simulink model "MySusp_FrcSystem_RTW"  (R2022a)
settings: Solver=ode1  StartTime=0.0  StopTime=inf  FixedStep=0.001  RelTol=1e-3
PreLoadFcn:
  | vehicle = 'Car'; if ~length(which('cmself')), cmenv; end
  | MySusp_FrcSystem_RTW_bus
  | MySusp_FrcSystem_RTW_params
InitFcn:
  | vehicle = 'Car'; if ~length(which('cmself')), cmenv; end
  | MySusp_FrcSystem_RTW_bus
undefined symbols (not defined in the file or in its folder): Damping_Pull_FL, Damping_Pull_FR, Damping_Pull_RL, Damping_Pull_RR, Damping_Push_FL, Damping_Push_FR, Damping_Push_RL, Damping_Push_RR, l0_Buffer_Pull_FL, l0_Buffer_Pull_FR, l0_Buffer_Pull_RL, l0_Buffer_Pull_RR, l0_Buffer_Push_FL, l0_Buffer_Push_FR, l0_Buffer_Push_RL, l0_Buffer_Push_RR, l0_Spring_FL, l0_Spring_FR, l0_Spring_RL, l0_Spring_RR, Stiffness_Buffer_Pull_FL, Stiffness_Buffer_Pull_FR, Stiffness_Buffer_Pull_RL, Stiffness_Buffer_Pull_RR, Stiffness_Buffer_Push_FL, Stiffness_Buffer_Push_FR, Stiffness_Buffer_Push_RL, Stiffness_Buffer_Push_RR, Stiffness_Spring_FL, Stiffness_Spring_FR, Stiffness_Spring_RL, Stiffness_Spring_RR, Stiffness_Stabi_F, Stiffness_Stabi_R
Description:
  | CarMaker Plug-in Model Target
settings Model: Creator=IPG  LastModifiedBy=IPG
settings SolverCC: AlgebraicLoopSolver=TrustRegion
settings DebuggingCC: UnconnectedInputMsg=warning  UnconnectedOutputMsg=warning  UnconnectedLineMsg=warning
settings RTWCC: Description=CarMaker Plug-in Model Target  SystemTargetFile=CarMaker.tlc  TemplateMakefile=CarMaker_unix-win64.tmf  DLArmComputeVersion=19.05
settings CodeAppCC: MaxIdLength=127
settings STFCustomTargetCC: TargetLangStandard=C99 (ISO)  CombineOutputUpdateFcns=on  CodeInterfacePackaging=Reusable function  GRTInterface=off  GenerateAllocFcn=on  SystemTargetFile=CarMaker.tlc
settings GRTTargetCC: ParMdlRefBuildCompliant=off  CompOptLevelCompliant=off  ConcurrentExecutionCompliant=off  MatFileLogging=off  CodeInterfacePackaging=Reusable function  CPPClassGenCompliant=off  GenerateAllocFcn=on  UseToolchainInfoCompliant=off

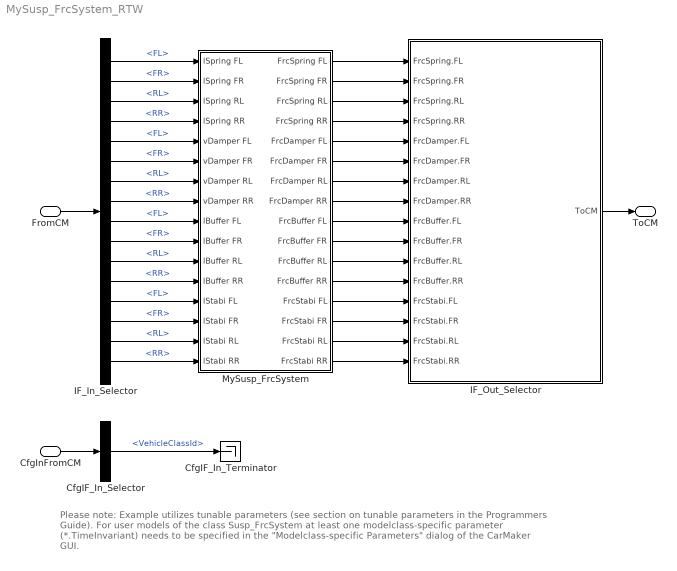
== system MySusp_FrcSystem_RTW ==
  note: Please note: Example utilizes tunable parameters (see section on tunable parameters in the Programmers Guide).
      |
      | For user models of the class Susp_FrcSystem at least one modelclass-specific parameter (*.TimeInvariant) needs to be
      | specified in the "Modelclass-specific Parameters" dialog of the CarMaker GUI.
  FromCM : Inport  OutDataTypeStr=Bus: cmSusp_FrcSystemIn
  CfgInFromCM : Inport  Port=2  OutDataTypeStr=Bus: cmSusp_FrcSystemCfgIn
  CfgIF_In_Selector : BusSelector  OutputSignals=VehicleClassId
  CfgIF_In_Terminator : Terminator
  IF_In_Selector : BusSelector  OutputSignals=lSpring.FL,lSpring.FR,lSpring.RL,lSpring.RR,vDamper.FL,vDamper.FR,vDamper.RL,vDamper.RR,lBuffer.FL,lBuffer.FR,lBuffer.RL,lBuffer.RR,lStabi.FL,lStabi.FR,lStabi.RL,lStabi.RR
  IF_Out_Selector : Subsystem  mask(Signal Selection){}
      mask help: Signal Selection Block
      settings: OpenFcn=cmSignalSelect('SignalSelection_CB',gcb)
  MySusp_FrcSystem : Subsystem
  ToCM : Outport  OutDataTypeStr=Bus: cmSusp_FrcSystemOut
  wires:
  FromCM/1 -> IF_In_Selector/1
  IF_Out_Selector/1(ToCM) -> ToCM/1
  CfgInFromCM/1 -> CfgIF_In_Selector/1
  CfgIF_In_Selector/1 -> CfgIF_In_Terminator/1  "<VehicleClassId>"
  MySusp_FrcSystem/1(FrcSpring FL) -> IF_Out_Selector/1(FrcSpring.FL)
  MySusp_FrcSystem/2(FrcSpring FR) -> IF_Out_Selector/2(FrcSpring.FR)
  MySusp_FrcSystem/3(FrcSpring RL) -> IF_Out_Selector/3(FrcSpring.RL)
  MySusp_FrcSystem/4(FrcSpring RR) -> IF_Out_Selector/4(FrcSpring.RR)
  MySusp_FrcSystem/5(FrcDamper FL) -> IF_Out_Selector/5(FrcDamper.FL)
  MySusp_FrcSystem/6(FrcDamper FR) -> IF_Out_Selector/6(FrcDamper.FR)
  MySusp_FrcSystem/7(FrcDamper RL) -> IF_Out_Selector/7(FrcDamper.RL)
  MySusp_FrcSystem/8(FrcDamper RR) -> IF_Out_Selector/8(FrcDamper.RR)
  MySusp_FrcSystem/9(FrcBuffer FL) -> IF_Out_Selector/9(FrcBuffer.FL)
  MySusp_FrcSystem/10(FrcBuffer FR) -> IF_Out_Selector/10(FrcBuffer.FR)
  MySusp_FrcSystem/11(FrcBuffer RL) -> IF_Out_Selector/11(FrcBuffer.RL)
  MySusp_FrcSystem/12(FrcBuffer RR) -> IF_Out_Selector/12(FrcBuffer.RR)
  MySusp_FrcSystem/13(FrcStabi FL) -> IF_Out_Selector/13(FrcStabi.FL)
  MySusp_FrcSystem/14(FrcStabi FR) -> IF_Out_Selector/14(FrcStabi.FR)
  MySusp_FrcSystem/15(FrcStabi RL) -> IF_Out_Selector/15(FrcStabi.RL)
  MySusp_FrcSystem/16(FrcStabi RR) -> IF_Out_Selector/16(FrcStabi.RR)
  IF_In_Selector/1 -> MySusp_FrcSystem/1(lSpring FL)  "<FL>"
  IF_In_Selector/2 -> MySusp_FrcSystem/2(lSpring FR)  "<FR>"
  IF_In_Selector/3 -> MySusp_FrcSystem/3(lSpring RL)  "<RL>"
  IF_In_Selector/4 -> MySusp_FrcSystem/4(lSpring RR)  "<RR>"
  IF_In_Selector/5 -> MySusp_FrcSystem/5(vDamper FL)  "<FL>"
  IF_In_Selector/6 -> MySusp_FrcSystem/6(vDamper FR)  "<FR>"
  IF_In_Selector/7 -> MySusp_FrcSystem/7(vDamper RL)  "<RL>"
  IF_In_Selector/8 -> MySusp_FrcSystem/8(vDamper RR)  "<RR>"
  IF_In_Selector/9 -> MySusp_FrcSystem/9(lBuffer FL)  "<FL>"
  IF_In_Selector/10 -> MySusp_FrcSystem/10(lBuffer FR)  "<FR>"
  IF_In_Selector/11 -> MySusp_FrcSystem/11(lBuffer RL)  "<RL>"
  IF_In_Selector/12 -> MySusp_FrcSystem/12(lBuffer RR)  "<RR>"
  IF_In_Selector/13 -> MySusp_FrcSystem/13(lStabi FL)  "<FL>"
  IF_In_Selector/14 -> MySusp_FrcSystem/14(lStabi FR)  "<FR>"
  IF_In_Selector/15 -> MySusp_FrcSystem/15(lStabi RL)  "<RL>"
  IF_In_Selector/16 -> MySusp_FrcSystem/16(lStabi RR)  "<RR>"

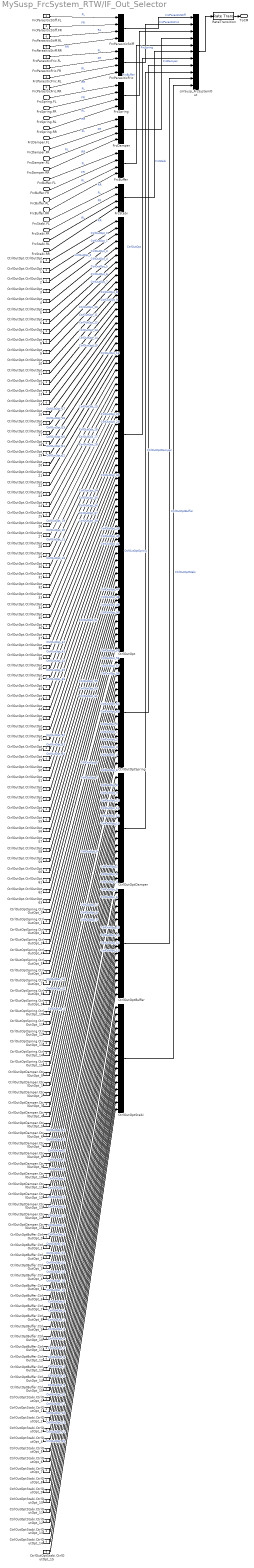
== system MySusp_FrcSystem_RTW/IF_Out_Selector ==
  FrcSpring.FL : Inport
  FrcSpring.FR : Inport  Port=2
  FrcSpring.RL : Inport  Port=3
  FrcSpring.RR : Inport  Port=4
  FrcDamper.FL : Inport  Port=5
  FrcDamper.FR : Inport  Port=6
  FrcDamper.RL : Inport  Port=7
  FrcDamper.RR : Inport  Port=8
  FrcBuffer.FL : Inport  Port=9
  FrcBuffer.FR : Inport  Port=10
  FrcBuffer.RL : Inport  Port=11
  FrcBuffer.RR : Inport  Port=12
  FrcStabi.FL : Inport  Port=13
  FrcStabi.FR : Inport  Port=14
  FrcStabi.RL : Inport  Port=15
  FrcStabi.RR : Inport  Port=16
  CtrlOutOpt : BusCreator  Inputs=64
  CtrlOutOpt.CtrlOutOpt_{0..63} (64 alike) : Constant  Value=0
  CtrlOutOptBuffer : BusCreator  Inputs=16
  CtrlOutOptBuffer.CtrlOutOpt_{0..15} (16 alike) : Constant  Value=0
  CtrlOutOptDamper : BusCreator  Inputs=16
  CtrlOutOptDamper.CtrlOutOpt_{0..15} (16 alike) : Constant  Value=0
  CtrlOutOptSpring : BusCreator  Inputs=16
  CtrlOutOptSpring.CtrlOutOpt_{0..15} (16 alike) : Constant  Value=0
  CtrlOutOptStabi : BusCreator  Inputs=16
  CtrlOutOptStabi.CtrlOutOpt_{0..15} (16 alike) : Constant  Value=0
  FrcBuffer : BusCreator  Inputs=4
  FrcDamper : BusCreator  Inputs=4
  FrcParasiticFric : BusCreator  Inputs=4
  FrcParasiticFric.FL : Constant  Value=0
  FrcParasiticFric.FR : Constant  Value=0
  FrcParasiticFric.RL : Constant  Value=0
  FrcParasiticFric.RR : Constant  Value=0
  FrcParasiticStiff : BusCreator  Inputs=4
  FrcParasiticStiff.FL : Constant  Value=0
  FrcParasiticStiff.FR : Constant  Value=0
  FrcParasiticStiff.RL : Constant  Value=0
  FrcParasiticStiff.RR : Constant  Value=0
  FrcSpring : BusCreator  Inputs=4
  FrcStabi : BusCreator  Inputs=4
  RateTransition : RateTransition  OutPortSampleTime=str2num(get_param(bdroot,'FixedStep'))
  cmSusp_FrcSystemOut : BusCreator  Inputs=11
  ToCM : Outport
  wires:
  RateTransition/1 -> ToCM/1
  cmSusp_FrcSystemOut/1 -> RateTransition/1
  FrcParasiticStiff/1 -> cmSusp_FrcSystemOut/1  "FrcParasiticStiff"
  FrcParasiticStiff.FL/1 -> FrcParasiticStiff/1  "FL"
  FrcParasiticStiff.FR/1 -> FrcParasiticStiff/2  "FR"
  FrcParasiticStiff.RL/1 -> FrcParasiticStiff/3  "RL"
  FrcParasiticStiff.RR/1 -> FrcParasiticStiff/4  "RR"
  FrcParasiticFric/1 -> cmSusp_FrcSystemOut/2  "FrcParasiticFric"
  FrcParasiticFric.FL/1 -> FrcParasiticFric/1  "FL"
  FrcParasiticFric.FR/1 -> FrcParasiticFric/2  "FR"
  FrcParasiticFric.RL/1 -> FrcParasiticFric/3  "RL"
  FrcParasiticFric.RR/1 -> FrcParasiticFric/4  "RR"
  FrcSpring/1 -> cmSusp_FrcSystemOut/3  "FrcSpring"
  FrcDamper/1 -> cmSusp_FrcSystemOut/4  "FrcDamper"
  FrcBuffer/1 -> cmSusp_FrcSystemOut/5  "FrcBuffer"
  FrcStabi/1 -> cmSusp_FrcSystemOut/6  "FrcStabi"
  CtrlOutOpt/1 -> cmSusp_FrcSystemOut/7  "CtrlOutOpt"
  CtrlOutOpt.CtrlOutOpt_0/1 -> CtrlOutOpt/1  "CtrlOutOpt_0"
  CtrlOutOpt.CtrlOutOpt_1/1 -> CtrlOutOpt/2  "CtrlOutOpt_1"
  CtrlOutOpt.CtrlOutOpt_2/1 -> CtrlOutOpt/3  "CtrlOutOpt_2"
  CtrlOutOpt.CtrlOutOpt_3/1 -> CtrlOutOpt/4  "CtrlOutOpt_3"
  CtrlOutOpt.CtrlOutOpt_4/1 -> CtrlOutOpt/5  "CtrlOutOpt_4"
  CtrlOutOpt.CtrlOutOpt_5/1 -> CtrlOutOpt/6  "CtrlOutOpt_5"
  CtrlOutOpt.CtrlOutOpt_6/1 -> CtrlOutOpt/7  "CtrlOutOpt_6"
  CtrlOutOpt.CtrlOutOpt_7/1 -> CtrlOutOpt/8  "CtrlOutOpt_7"
  CtrlOutOpt.CtrlOutOpt_8/1 -> CtrlOutOpt/9  "CtrlOutOpt_8"
  CtrlOutOpt.CtrlOutOpt_9/1 -> CtrlOutOpt/10  "CtrlOutOpt_9"
  CtrlOutOpt.CtrlOutOpt_10/1 -> CtrlOutOpt/11  "CtrlOutOpt_10"
  CtrlOutOpt.CtrlOutOpt_11/1 -> CtrlOutOpt/12  "CtrlOutOpt_11"
  CtrlOutOpt.CtrlOutOpt_12/1 -> CtrlOutOpt/13  "CtrlOutOpt_12"
  CtrlOutOpt.CtrlOutOpt_13/1 -> CtrlOutOpt/14  "CtrlOutOpt_13"
  CtrlOutOpt.CtrlOutOpt_14/1 -> CtrlOutOpt/15  "CtrlOutOpt_14"
  CtrlOutOpt.CtrlOutOpt_15/1 -> CtrlOutOpt/16  "CtrlOutOpt_15"
  CtrlOutOpt.CtrlOutOpt_16/1 -> CtrlOutOpt/17  "CtrlOutOpt_16"
  CtrlOutOpt.CtrlOutOpt_17/1 -> CtrlOutOpt/18  "CtrlOutOpt_17"
  CtrlOutOpt.CtrlOutOpt_18/1 -> CtrlOutOpt/19  "CtrlOutOpt_18"
  CtrlOutOpt.CtrlOutOpt_19/1 -> CtrlOutOpt/20  "CtrlOutOpt_19"
  CtrlOutOpt.CtrlOutOpt_20/1 -> CtrlOutOpt/21  "CtrlOutOpt_20"
  CtrlOutOpt.CtrlOutOpt_21/1 -> CtrlOutOpt/22  "CtrlOutOpt_21"
  CtrlOutOpt.CtrlOutOpt_22/1 -> CtrlOutOpt/23  "CtrlOutOpt_22"
  CtrlOutOpt.CtrlOutOpt_23/1 -> CtrlOutOpt/24  "CtrlOutOpt_23"
  CtrlOutOpt.CtrlOutOpt_24/1 -> CtrlOutOpt/25  "CtrlOutOpt_24"
  CtrlOutOpt.CtrlOutOpt_25/1 -> CtrlOutOpt/26  "CtrlOutOpt_25"
  CtrlOutOpt.CtrlOutOpt_26/1 -> CtrlOutOpt/27  "CtrlOutOpt_26"
  CtrlOutOpt.CtrlOutOpt_27/1 -> CtrlOutOpt/28  "CtrlOutOpt_27"
  CtrlOutOpt.CtrlOutOpt_28/1 -> CtrlOutOpt/29  "CtrlOutOpt_28"
  CtrlOutOpt.CtrlOutOpt_29/1 -> CtrlOutOpt/30  "CtrlOutOpt_29"
  CtrlOutOpt.CtrlOutOpt_30/1 -> CtrlOutOpt/31  "CtrlOutOpt_30"
  CtrlOutOpt.CtrlOutOpt_31/1 -> CtrlOutOpt/32  "CtrlOutOpt_31"
  CtrlOutOpt.CtrlOutOpt_32/1 -> CtrlOutOpt/33  "CtrlOutOpt_32"
  CtrlOutOpt.CtrlOutOpt_33/1 -> CtrlOutOpt/34  "CtrlOutOpt_33"
  CtrlOutOpt.CtrlOutOpt_34/1 -> CtrlOutOpt/35  "CtrlOutOpt_34"
  CtrlOutOpt.CtrlOutOpt_35/1 -> CtrlOutOpt/36  "CtrlOutOpt_35"
  CtrlOutOpt.CtrlOutOpt_36/1 -> CtrlOutOpt/37  "CtrlOutOpt_36"
  CtrlOutOpt.CtrlOutOpt_37/1 -> CtrlOutOpt/38  "CtrlOutOpt_37"
  CtrlOutOpt.CtrlOutOpt_38/1 -> CtrlOutOpt/39  "CtrlOutOpt_38"
  CtrlOutOpt.CtrlOutOpt_39/1 -> CtrlOutOpt/40  "CtrlOutOpt_39"
  CtrlOutOpt.CtrlOutOpt_40/1 -> CtrlOutOpt/41  "CtrlOutOpt_40"
  CtrlOutOpt.CtrlOutOpt_41/1 -> CtrlOutOpt/42  "CtrlOutOpt_41"
  CtrlOutOpt.CtrlOutOpt_42/1 -> CtrlOutOpt/43  "CtrlOutOpt_42"
  CtrlOutOpt.CtrlOutOpt_43/1 -> CtrlOutOpt/44  "CtrlOutOpt_43"
  CtrlOutOpt.CtrlOutOpt_44/1 -> CtrlOutOpt/45  "CtrlOutOpt_44"
  CtrlOutOpt.CtrlOutOpt_45/1 -> CtrlOutOpt/46  "CtrlOutOpt_45"
  CtrlOutOpt.CtrlOutOpt_46/1 -> CtrlOutOpt/47  "CtrlOutOpt_46"
  CtrlOutOpt.CtrlOutOpt_47/1 -> CtrlOutOpt/48  "CtrlOutOpt_47"
  CtrlOutOpt.CtrlOutOpt_48/1 -> CtrlOutOpt/49  "CtrlOutOpt_48"
  CtrlOutOpt.CtrlOutOpt_49/1 -> CtrlOutOpt/50  "CtrlOutOpt_49"
  CtrlOutOpt.CtrlOutOpt_50/1 -> CtrlOutOpt/51  "CtrlOutOpt_50"
  CtrlOutOpt.CtrlOutOpt_51/1 -> CtrlOutOpt/52  "CtrlOutOpt_51"
  CtrlOutOpt.CtrlOutOpt_52/1 -> CtrlOutOpt/53  "CtrlOutOpt_52"
  CtrlOutOpt.CtrlOutOpt_53/1 -> CtrlOutOpt/54  "CtrlOutOpt_53"
  CtrlOutOpt.CtrlOutOpt_54/1 -> CtrlOutOpt/55  "CtrlOutOpt_54"
  CtrlOutOpt.CtrlOutOpt_55/1 -> CtrlOutOpt/56  "CtrlOutOpt_55"
  CtrlOutOpt.CtrlOutOpt_56/1 -> CtrlOutOpt/57  "CtrlOutOpt_56"
  CtrlOutOpt.CtrlOutOpt_57/1 -> CtrlOutOpt/58  "CtrlOutOpt_57"
  CtrlOutOpt.CtrlOutOpt_58/1 -> CtrlOutOpt/59  "CtrlOutOpt_58"
  CtrlOutOpt.CtrlOutOpt_59/1 -> CtrlOutOpt/60  "CtrlOutOpt_59"
  CtrlOutOpt.CtrlOutOpt_60/1 -> CtrlOutOpt/61  "CtrlOutOpt_60"
  CtrlOutOpt.CtrlOutOpt_61/1 -> CtrlOutOpt/62  "CtrlOutOpt_61"
  CtrlOutOpt.CtrlOutOpt_62/1 -> CtrlOutOpt/63  "CtrlOutOpt_62"
  CtrlOutOpt.CtrlOutOpt_63/1 -> CtrlOutOpt/64  "CtrlOutOpt_63"
  CtrlOutOptSpring/1 -> cmSusp_FrcSystemOut/8  "CtrlOutOptSpring"
  CtrlOutOptSpring.CtrlOutOpt_0/1 -> CtrlOutOptSpring/1  "CtrlOutOpt_0"
  CtrlOutOptSpring.CtrlOutOpt_1/1 -> CtrlOutOptSpring/2  "CtrlOutOpt_1"
  CtrlOutOptSpring.CtrlOutOpt_2/1 -> CtrlOutOptSpring/3  "CtrlOutOpt_2"
  CtrlOutOptSpring.CtrlOutOpt_3/1 -> CtrlOutOptSpring/4  "CtrlOutOpt_3"
  CtrlOutOptSpring.CtrlOutOpt_4/1 -> CtrlOutOptSpring/5  "CtrlOutOpt_4"
  CtrlOutOptSpring.CtrlOutOpt_5/1 -> CtrlOutOptSpring/6  "CtrlOutOpt_5"
  CtrlOutOptSpring.CtrlOutOpt_6/1 -> CtrlOutOptSpring/7  "CtrlOutOpt_6"
  CtrlOutOptSpring.CtrlOutOpt_7/1 -> CtrlOutOptSpring/8  "CtrlOutOpt_7"
  CtrlOutOptSpring.CtrlOutOpt_8/1 -> CtrlOutOptSpring/9  "CtrlOutOpt_8"
  CtrlOutOptSpring.CtrlOutOpt_9/1 -> CtrlOutOptSpring/10  "CtrlOutOpt_9"
  CtrlOutOptSpring.CtrlOutOpt_10/1 -> CtrlOutOptSpring/11  "CtrlOutOpt_10"
  CtrlOutOptSpring.CtrlOutOpt_11/1 -> CtrlOutOptSpring/12  "CtrlOutOpt_11"
  CtrlOutOptSpring.CtrlOutOpt_12/1 -> CtrlOutOptSpring/13  "CtrlOutOpt_12"
  CtrlOutOptSpring.CtrlOutOpt_13/1 -> CtrlOutOptSpring/14  "CtrlOutOpt_13"
  CtrlOutOptSpring.CtrlOutOpt_14/1 -> CtrlOutOptSpring/15  "CtrlOutOpt_14"
  CtrlOutOptSpring.CtrlOutOpt_15/1 -> CtrlOutOptSpring/16  "CtrlOutOpt_15"
  CtrlOutOptDamper/1 -> cmSusp_FrcSystemOut/9  "CtrlOutOptDamper"
  CtrlOutOptDamper.CtrlOutOpt_0/1 -> CtrlOutOptDamper/1  "CtrlOutOpt_0"
  CtrlOutOptDamper.CtrlOutOpt_1/1 -> CtrlOutOptDamper/2  "CtrlOutOpt_1"
  CtrlOutOptDamper.CtrlOutOpt_2/1 -> CtrlOutOptDamper/3  "CtrlOutOpt_2"
  CtrlOutOptDamper.CtrlOutOpt_3/1 -> CtrlOutOptDamper/4  "CtrlOutOpt_3"
  CtrlOutOptDamper.CtrlOutOpt_4/1 -> CtrlOutOptDamper/5  "CtrlOutOpt_4"
  CtrlOutOptDamper.CtrlOutOpt_5/1 -> CtrlOutOptDamper/6  "CtrlOutOpt_5"
  CtrlOutOptDamper.CtrlOutOpt_6/1 -> CtrlOutOptDamper/7  "CtrlOutOpt_6"
  CtrlOutOptDamper.CtrlOutOpt_7/1 -> CtrlOutOptDamper/8  "CtrlOutOpt_7"
  CtrlOutOptDamper.CtrlOutOpt_8/1 -> CtrlOutOptDamper/9  "CtrlOutOpt_8"
  CtrlOutOptDamper.CtrlOutOpt_9/1 -> CtrlOutOptDamper/10  "CtrlOutOpt_9"
  CtrlOutOptDamper.CtrlOutOpt_10/1 -> CtrlOutOptDamper/11  "CtrlOutOpt_10"
  CtrlOutOptDamper.CtrlOutOpt_11/1 -> CtrlOutOptDamper/12  "CtrlOutOpt_11"
  CtrlOutOptDamper.CtrlOutOpt_12/1 -> CtrlOutOptDamper/13  "CtrlOutOpt_12"
  CtrlOutOptDamper.CtrlOutOpt_13/1 -> CtrlOutOptDamper/14  "CtrlOutOpt_13"
  CtrlOutOptDamper.CtrlOutOpt_14/1 -> CtrlOutOptDamper/15  "CtrlOutOpt_14"
  CtrlOutOptDamper.CtrlOutOpt_15/1 -> CtrlOutOptDamper/16  "CtrlOutOpt_15"
  CtrlOutOptBuffer/1 -> cmSusp_FrcSystemOut/10  "CtrlOutOptBuffer"
  CtrlOutOptBuffer.CtrlOutOpt_0/1 -> CtrlOutOptBuffer/1  "CtrlOutOpt_0"
  CtrlOutOptBuffer.CtrlOutOpt_1/1 -> CtrlOutOptBuffer/2  "CtrlOutOpt_1"
  CtrlOutOptBuffer.CtrlOutOpt_2/1 -> CtrlOutOptBuffer/3  "CtrlOutOpt_2"
  CtrlOutOptBuffer.CtrlOutOpt_3/1 -> CtrlOutOptBuffer/4  "CtrlOutOpt_3"
  CtrlOutOptBuffer.CtrlOutOpt_4/1 -> CtrlOutOptBuffer/5  "CtrlOutOpt_4"
  CtrlOutOptBuffer.CtrlOutOpt_5/1 -> CtrlOutOptBuffer/6  "CtrlOutOpt_5"
  CtrlOutOptBuffer.CtrlOutOpt_6/1 -> CtrlOutOptBuffer/7  "CtrlOutOpt_6"
  CtrlOutOptBuffer.CtrlOutOpt_7/1 -> CtrlOutOptBuffer/8  "CtrlOutOpt_7"
  CtrlOutOptBuffer.CtrlOutOpt_8/1 -> CtrlOutOptBuffer/9  "CtrlOutOpt_8"
  CtrlOutOptBuffer.CtrlOutOpt_9/1 -> CtrlOutOptBuffer/10  "CtrlOutOpt_9"
  CtrlOutOptBuffer.CtrlOutOpt_10/1 -> CtrlOutOptBuffer/11  "CtrlOutOpt_10"
  CtrlOutOptBuffer.CtrlOutOpt_11/1 -> CtrlOutOptBuffer/12  "CtrlOutOpt_11"
  CtrlOutOptBuffer.CtrlOutOpt_12/1 -> CtrlOutOptBuffer/13  "CtrlOutOpt_12"
  CtrlOutOptBuffer.CtrlOutOpt_13/1 -> CtrlOutOptBuffer/14  "CtrlOutOpt_13"
  CtrlOutOptBuffer.CtrlOutOpt_14/1 -> CtrlOutOptBuffer/15  "CtrlOutOpt_14"
  CtrlOutOptBuffer.CtrlOutOpt_15/1 -> CtrlOutOptBuffer/16  "CtrlOutOpt_15"
  CtrlOutOptStabi/1 -> cmSusp_FrcSystemOut/11  "CtrlOutOptStabi"
  CtrlOutOptStabi.CtrlOutOpt_0/1 -> CtrlOutOptStabi/1  "CtrlOutOpt_0"
  CtrlOutOptStabi.CtrlOutOpt_1/1 -> CtrlOutOptStabi/2  "CtrlOutOpt_1"
  CtrlOutOptStabi.CtrlOutOpt_2/1 -> CtrlOutOptStabi/3  "CtrlOutOpt_2"
  CtrlOutOptStabi.CtrlOutOpt_3/1 -> CtrlOutOptStabi/4  "CtrlOutOpt_3"
  CtrlOutOptStabi.CtrlOutOpt_4/1 -> CtrlOutOptStabi/5  "CtrlOutOpt_4"
  CtrlOutOptStabi.CtrlOutOpt_5/1 -> CtrlOutOptStabi/6  "CtrlOutOpt_5"
  CtrlOutOptStabi.CtrlOutOpt_6/1 -> CtrlOutOptStabi/7  "CtrlOutOpt_6"
  CtrlOutOptStabi.CtrlOutOpt_7/1 -> CtrlOutOptStabi/8  "CtrlOutOpt_7"
  CtrlOutOptStabi.CtrlOutOpt_8/1 -> CtrlOutOptStabi/9  "CtrlOutOpt_8"
  CtrlOutOptStabi.CtrlOutOpt_9/1 -> CtrlOutOptStabi/10  "CtrlOutOpt_9"
  CtrlOutOptStabi.CtrlOutOpt_10/1 -> CtrlOutOptStabi/11  "CtrlOutOpt_10"
  CtrlOutOptStabi.CtrlOutOpt_11/1 -> CtrlOutOptStabi/12  "CtrlOutOpt_11"
  CtrlOutOptStabi.CtrlOutOpt_12/1 -> CtrlOutOptStabi/13  "CtrlOutOpt_12"
  CtrlOutOptStabi.CtrlOutOpt_13/1 -> CtrlOutOptStabi/14  "CtrlOutOpt_13"
  CtrlOutOptStabi.CtrlOutOpt_14/1 -> CtrlOutOptStabi/15  "CtrlOutOpt_14"
  CtrlOutOptStabi.CtrlOutOpt_15/1 -> CtrlOutOptStabi/16  "CtrlOutOpt_15"
  FrcSpring.FL/1 -> FrcSpring/1  "FL"
  FrcSpring.FR/1 -> FrcSpring/2  "FR"
  FrcSpring.RL/1 -> FrcSpring/3  "RL"
  FrcSpring.RR/1 -> FrcSpring/4  "RR"
  FrcDamper.FL/1 -> FrcDamper/1  "FL"
  FrcDamper.FR/1 -> FrcDamper/2  "FR"
  FrcDamper.RL/1 -> FrcDamper/3  "RL"
  FrcDamper.RR/1 -> FrcDamper/4  "RR"
  FrcBuffer.FL/1 -> FrcBuffer/1  "FL"
  FrcBuffer.FR/1 -> FrcBuffer/2  "FR"
  FrcBuffer.RL/1 -> FrcBuffer/3  "RL"
  FrcBuffer.RR/1 -> FrcBuffer/4  "RR"
  FrcStabi.FL/1 -> FrcStabi/1  "FL"
  FrcStabi.FR/1 -> FrcStabi/2  "FR"
  FrcStabi.RL/1 -> FrcStabi/3  "RL"
  FrcStabi.RR/1 -> FrcStabi/4  "RR"

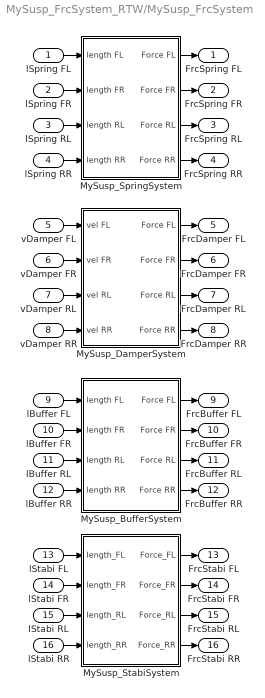
== system MySusp_FrcSystem_RTW/MySusp_FrcSystem ==
  lSpring FL : Inport
  lSpring FR : Inport  Port=2
  lSpring RL : Inport  Port=3
  lSpring RR : Inport  Port=4
  vDamper FL : Inport  Port=5
  vDamper FR : Inport  Port=6
  vDamper RL : Inport  Port=7
  vDamper RR : Inport  Port=8
  lBuffer FL : Inport  Port=9
  lBuffer FR : Inport  Port=10
  lBuffer RL : Inport  Port=11
  lBuffer RR : Inport  Port=12
  lStabi FL : Inport  Port=13
  lStabi FR : Inport  Port=14
  lStabi RL : Inport  Port=15
  lStabi RR : Inport  Port=16
  MySusp_BufferSystem : Subsystem
  MySusp_DamperSystem : Subsystem
  MySusp_SpringSystem : Subsystem
  MySusp_StabiSystem : Subsystem
  FrcSpring FL : Outport
  FrcSpring FR : Outport  Port=2
  FrcSpring RL : Outport  Port=3
  FrcSpring RR : Outport  Port=4
  FrcDamper FL : Outport  Port=5
  FrcDamper FR : Outport  Port=6
  FrcDamper RL : Outport  Port=7
  FrcDamper RR : Outport  Port=8
  FrcBuffer FL : Outport  Port=9
  FrcBuffer FR : Outport  Port=10
  FrcBuffer RL : Outport  Port=11
  FrcBuffer RR : Outport  Port=12
  FrcStabi FL : Outport  Port=13
  FrcStabi FR : Outport  Port=14
  FrcStabi RL : Outport  Port=15
  FrcStabi RR : Outport  Port=16
  wires:
  MySusp_SpringSystem/1(Force FL) -> FrcSpring FL/1
  lStabi RR/1 -> MySusp_StabiSystem/4(length_RR)
  lStabi RL/1 -> MySusp_StabiSystem/3(Iength_RL)
  MySusp_StabiSystem/3(Force_RL) -> FrcStabi RL/1
  lBuffer RL/1 -> MySusp_BufferSystem/3(length RL)
  MySusp_StabiSystem/2(Force_FR) -> FrcStabi FR/1
  MySusp_DamperSystem/2(Force FR) -> FrcDamper FR/1
  MySusp_BufferSystem/1(Force FL) -> FrcBuffer FL/1
  vDamper RL/1 -> MySusp_DamperSystem/3(vel RL)
  MySusp_StabiSystem/1(Force_FL) -> FrcStabi FL/1
  MySusp_SpringSystem/4(Force RR) -> FrcSpring RR/1
  MySusp_DamperSystem/4(Force RR) -> FrcDamper RR/1
  lSpring FL/1 -> MySusp_SpringSystem/1(length FL)
  MySusp_DamperSystem/1(Force FL) -> FrcDamper FL/1
  MySusp_BufferSystem/2(Force FR) -> FrcBuffer FR/1
  MySusp_SpringSystem/2(Force FR) -> FrcSpring FR/1
  lBuffer FL/1 -> MySusp_BufferSystem/1(length FL)
  MySusp_StabiSystem/4(Force_RR) -> FrcStabi RR/1
  vDamper RR/1 -> MySusp_DamperSystem/4(vel RR)
  vDamper FL/1 -> MySusp_DamperSystem/1(vel FL)
  lStabi FR/1 -> MySusp_StabiSystem/2(length_FR)
  MySusp_DamperSystem/3(Force RL) -> FrcDamper RL/1
  lBuffer FR/1 -> MySusp_BufferSystem/2(length FR)
  vDamper FR/1 -> MySusp_DamperSystem/2(vel FR)
  MySusp_BufferSystem/3(Force RL) -> FrcBuffer RL/1
  MySusp_BufferSystem/4(Force RR) -> FrcBuffer RR/1
  MySusp_SpringSystem/3(Force RL) -> FrcSpring RL/1
  lSpring FR/1 -> MySusp_SpringSystem/2(length FR)
  lSpring RL/1 -> MySusp_SpringSystem/3(length RL)
  lSpring RR/1 -> MySusp_SpringSystem/4(length RR)
  lBuffer RR/1 -> MySusp_BufferSystem/4(length RR)
  lStabi FL/1 -> MySusp_StabiSystem/1(Iength_FL)

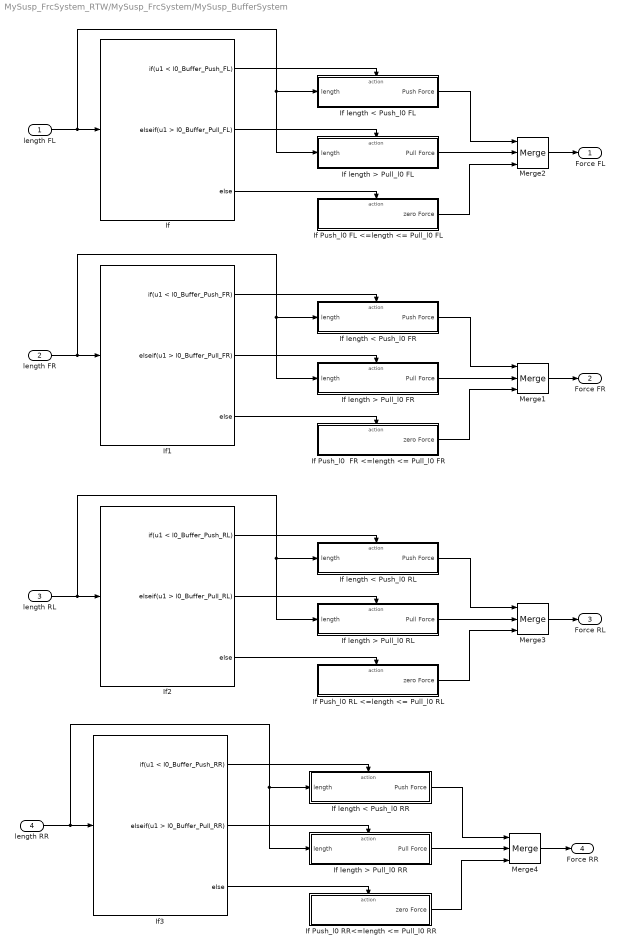
== system MySusp_FrcSystem_RTW/MySusp_FrcSystem/MySusp_BufferSystem ==
  length FL : Inport
  length FR : Inport  Port=2
  length RL : Inport  Port=3
  length RR : Inport  Port=4
  If : If  IfExpression=u1 < l0_Buffer_Push_FL  ElseIfExpressions=u1 > l0_Buffer_Pull_FL
  If Push_l0  FR <=length <= Pull_l0 FR : Subsystem  TreatAsAtomicUnit=on
  "If Push_l0 FL <=length <= Pull_l0 FL " : Subsystem  TreatAsAtomicUnit=on
  If Push_l0 RL <=length <= Pull_l0 RL : Subsystem  TreatAsAtomicUnit=on
  If Push_l0 RR<=length <= Pull_l0 RR : Subsystem  TreatAsAtomicUnit=on
  If length < Push_l0 FL : Subsystem  TreatAsAtomicUnit=on
  If length < Push_l0 FR : Subsystem  TreatAsAtomicUnit=on
  If length < Push_l0 RL : Subsystem  TreatAsAtomicUnit=on
  If length < Push_l0 RR : Subsystem  TreatAsAtomicUnit=on
  If length > Pull_l0 FL : Subsystem  TreatAsAtomicUnit=on
  If length > Pull_l0 FR : Subsystem  TreatAsAtomicUnit=on
  If length > Pull_l0 RL : Subsystem  TreatAsAtomicUnit=on
  If length > Pull_l0 RR : Subsystem  TreatAsAtomicUnit=on
  If1 : If  IfExpression=u1 < l0_Buffer_Push_FR  ElseIfExpressions=u1 > l0_Buffer_Pull_FR
  If2 : If  IfExpression=u1 < l0_Buffer_Push_RL  ElseIfExpressions=u1 > l0_Buffer_Pull_RL
  If3 : If  IfExpression=u1 < l0_Buffer_Push_RR  ElseIfExpressions=u1 > l0_Buffer_Pull_RR
  Merge{1..4} (4 alike) : Merge  Inputs=3
  Force FL : Outport  VectorParamsAs1DForOutWhenUnconnected=off
  Force FR : Outport  Port=2  VectorParamsAs1DForOutWhenUnconnected=off
  Force RL : Outport  Port=3  VectorParamsAs1DForOutWhenUnconnected=off
  Force RR : Outport  Port=4  VectorParamsAs1DForOutWhenUnconnected=off
  wires:
  length FL/1 -> If length > Pull_l0 FL/1(length), If length < Push_l0 FL/1(length), If/1
  If/3 -> "If Push_l0 FL <=length <= Pull_l0 FL "/Action
  If/2 -> If length > Pull_l0 FL/Action
  If/1 -> If length < Push_l0 FL/Action
  If length < Push_l0 FL/1(Push Force) -> Merge2/1
  "If Push_l0 FL <=length <= Pull_l0 FL "/1(zero Force) -> Merge2/3
  If length > Pull_l0 FL/1(Pull Force) -> Merge2/2
  Merge2/1 -> Force FL/1
  If Push_l0  FR <=length <= Pull_l0 FR/1(zero Force) -> Merge1/3
  If length > Pull_l0 FR/1(Pull Force) -> Merge1/2
  If1/1 -> If length < Push_l0 FR/Action
  length FR/1 -> If length > Pull_l0 FR/1(length), If length < Push_l0 FR/1(length), If1/1
  If1/2 -> If length > Pull_l0 FR/Action
  If1/3 -> If Push_l0  FR <=length <= Pull_l0 FR/Action
  Merge1/1 -> Force FR/1
  If length < Push_l0 FR/1(Push Force) -> Merge1/1
  If Push_l0 RL <=length <= Pull_l0 RL/1(zero Force) -> Merge3/3
  If length > Pull_l0 RL/1(Pull Force) -> Merge3/2
  If2/1 -> If length < Push_l0 RL/Action
  length RL/1 -> If length > Pull_l0 RL/1(length), If length < Push_l0 RL/1(length), If2/1
  If2/2 -> If length > Pull_l0 RL/Action
  If2/3 -> If Push_l0 RL <=length <= Pull_l0 RL/Action
  Merge3/1 -> Force RL/1
  If length < Push_l0 RL/1(Push Force) -> Merge3/1
  If Push_l0 RR<=length <= Pull_l0 RR/1(zero Force) -> Merge4/3
  If length > Pull_l0 RR/1(Pull Force) -> Merge4/2
  If3/1 -> If length < Push_l0 RR/Action
  length RR/1 -> If length > Pull_l0 RR/1(length), If length < Push_l0 RR/1(length), If3/1
  If3/2 -> If length > Pull_l0 RR/Action
  If3/3 -> If Push_l0 RR<=length <= Pull_l0 RR/Action
  Merge4/1 -> Force RR/1
  If length < Push_l0 RR/1(Push Force) -> Merge4/1

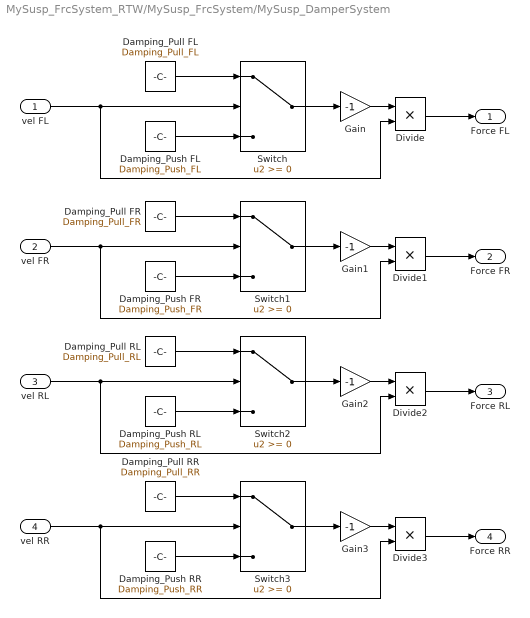
== system MySusp_FrcSystem_RTW/MySusp_FrcSystem/MySusp_DamperSystem ==
  vel FL : Inport
  vel FR : Inport  Port=2
  vel RL : Inport  Port=3
  vel RR : Inport  Port=4
  Damping_Pull FL : Constant  Value=Damping_Pull_FL
  Damping_Pull FR : Constant  Value=Damping_Pull_FR
  Damping_Pull RL : Constant  Value=Damping_Pull_RL
  Damping_Pull RR : Constant  Value=Damping_Pull_RR
  Damping_Push FL : Constant  Value=Damping_Push_FL
  Damping_Push FR : Constant  Value=Damping_Push_FR
  Damping_Push RL : Constant  Value=Damping_Push_RL
  Damping_Push RR : Constant  Value=Damping_Push_RR
  Divide{,1..3} (4 alike) : Product  Inputs=**
  Gain{,1..3} (4 alike) : Gain  Gain=-1
  Switch{,1..3} (4 alike) : Switch  SaturateOnIntegerOverflow=off  InputSameDT=off
  Force FL : Outport  VectorParamsAs1DForOutWhenUnconnected=off
  Force FR : Outport  Port=2  VectorParamsAs1DForOutWhenUnconnected=off
  Force RL : Outport  Port=3  VectorParamsAs1DForOutWhenUnconnected=off
  Force RR : Outport  Port=4  VectorParamsAs1DForOutWhenUnconnected=off
  wires:
  vel FL/1 -> Divide/2, Switch/2
  Switch/1 -> Gain/1
  Damping_Pull FL/1 -> Switch/1
  Damping_Push FL/1 -> Switch/3
  Gain/1 -> Divide/1
  Divide/1 -> Force FL/1
  Gain1/1 -> Divide1/1
  vel FR/1 -> Divide1/2, Switch1/2
  Switch1/1 -> Gain1/1
  Divide1/1 -> Force FR/1
  Damping_Pull FR/1 -> Switch1/1
  Damping_Push FR/1 -> Switch1/3
  Damping_Push RL/1 -> Switch2/3
  vel RL/1 -> Divide2/2, Switch2/2
  Damping_Pull RL/1 -> Switch2/1
  Switch2/1 -> Gain2/1
  Divide2/1 -> Force RL/1
  Gain2/1 -> Divide2/1
  Damping_Push RR/1 -> Switch3/3
  vel RR/1 -> Divide3/2, Switch3/2
  Damping_Pull RR/1 -> Switch3/1
  Switch3/1 -> Gain3/1
  Divide3/1 -> Force RR/1
  Gain3/1 -> Divide3/1

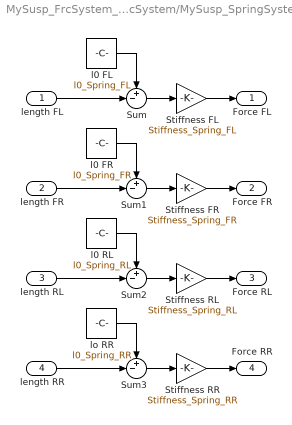
== system MySusp_FrcSystem_RTW/MySusp_FrcSystem/MySusp_SpringSystem ==
  length FL : Inport
  length FR : Inport  Port=2
  length RL : Inport  Port=3
  length RR : Inport  Port=4
  Stiffness FL : Gain  Gain=Stiffness_Spring_FL
  Stiffness FR : Gain  Gain=Stiffness_Spring_FR
  Stiffness RL : Gain  Gain=Stiffness_Spring_RL
  Stiffness RR : Gain  Gain=Stiffness_Spring_RR
  Sum{,1..3} (4 alike) : Sum  Inputs=+-|
  l0 FL : Constant  Value=l0_Spring_FL
  l0 FR : Constant  Value=l0_Spring_FR
  l0 RL : Constant  Value=l0_Spring_RL
  lo RR : Constant  Value=l0_Spring_RR
  Force FL : Outport  VectorParamsAs1DForOutWhenUnconnected=off
  Force FR : Outport  Port=2  VectorParamsAs1DForOutWhenUnconnected=off
  Force RL : Outport  Port=3  VectorParamsAs1DForOutWhenUnconnected=off
  Force RR : Outport  Port=4  VectorParamsAs1DForOutWhenUnconnected=off
  wires:
  length FL/1 -> Sum/2
  Stiffness FL/1 -> Force FL/1
  l0 FL/1 -> Sum/1
  Sum/1 -> Stiffness FL/1
  Stiffness FR/1 -> Force FR/1
  length FR/1 -> Sum1/2
  l0 FR/1 -> Sum1/1
  Sum1/1 -> Stiffness FR/1
  Stiffness RL/1 -> Force RL/1
  length RL/1 -> Sum2/2
  l0 RL/1 -> Sum2/1
  Sum2/1 -> Stiffness RL/1
  Stiffness RR/1 -> Force RR/1
  length RR/1 -> Sum3/2
  lo RR/1 -> Sum3/1
  Sum3/1 -> Stiffness RR/1

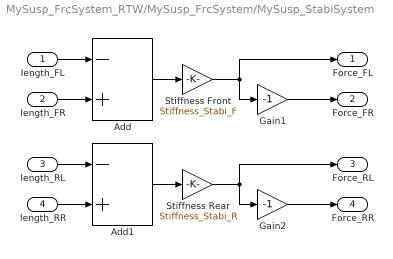
== system MySusp_FrcSystem_RTW/MySusp_FrcSystem/MySusp_StabiSystem ==
  Iength_FL : Inport
  length_FR : Inport  Port=2
  Iength_RL : Inport  Port=3
  length_RR : Inport  Port=4
  Add : Sum  Inputs=-+
  Add1 : Sum  Inputs=-+
  Gain1 : Gain  Gain=-1
  Gain2 : Gain  Gain=-1
  Stiffness Front : Gain  Gain=Stiffness_Stabi_F
  Stiffness Rear : Gain  Gain=Stiffness_Stabi_R
  Force_FL : Outport  VectorParamsAs1DForOutWhenUnconnected=off
  Force_FR : Outport  Port=2  VectorParamsAs1DForOutWhenUnconnected=off
  Force_RL : Outport  Port=3  VectorParamsAs1DForOutWhenUnconnected=off
  Force_RR : Outport  Port=4  VectorParamsAs1DForOutWhenUnconnected=off
  wires:
  Stiffness Front/1 -> Force_FL/1, Gain1/1
  Gain1/1 -> Force_FR/1
  Iength_FL/1 -> Add/1
  length_FR/1 -> Add/2
  Add/1 -> Stiffness Front/1
  Gain2/1 -> Force_RR/1
  Add1/1 -> Stiffness Rear/1
  Stiffness Rear/1 -> Force_RL/1, Gain2/1
  Iength_RL/1 -> Add1/1
  length_RR/1 -> Add1/2

== system MySusp_FrcSystem_RTW/MySusp_FrcSystem/MySusp_BufferSystem/If Push_l0  FR <=length <= Pull_l0 FR ==
  length < Push_l0 : ActionPort  ActionPortLabel=else
  Constant : Constant  Value=0.0
  zero Force : Outport  InitialOutput=0  VectorParamsAs1DForOutWhenUnconnected=off
  wires:
  Constant/1 -> zero Force/1

== system MySusp_FrcSystem_RTW/MySusp_FrcSystem/MySusp_BufferSystem/If Push_l0 FL <=length <= Pull_l0 FL  ==
  length < Push_l0 : ActionPort  ActionPortLabel=else
  Constant : Constant  Value=0.0
  zero Force : Outport  InitialOutput=0  VectorParamsAs1DForOutWhenUnconnected=off
  wires:
  Constant/1 -> zero Force/1

== system MySusp_FrcSystem_RTW/MySusp_FrcSystem/MySusp_BufferSystem/If Push_l0 RL <=length <= Pull_l0 RL ==
  length < Push_l0 : ActionPort  ActionPortLabel=else
  Constant : Constant  Value=0.0
  zero Force : Outport  InitialOutput=0  VectorParamsAs1DForOutWhenUnconnected=off
  wires:
  Constant/1 -> zero Force/1

== system MySusp_FrcSystem_RTW/MySusp_FrcSystem/MySusp_BufferSystem/If Push_l0 RR<=length <= Pull_l0 RR ==
  length < Push_l0 : ActionPort  ActionPortLabel=else
  Constant : Constant  Value=0.0
  zero Force : Outport  InitialOutput=0  VectorParamsAs1DForOutWhenUnconnected=off
  wires:
  Constant/1 -> zero Force/1

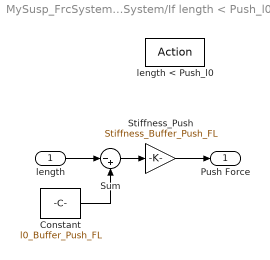
== system MySusp_FrcSystem_RTW/MySusp_FrcSystem/MySusp_BufferSystem/If length < Push_l0 FL ==
  length : Inport
  length < Push_l0 : ActionPort  ActionPortLabel=if(u1 < l0_Buffer_Push_FL)
  Constant : Constant  Value=l0_Buffer_Push_FL
  Stiffness_Push : Gain  Gain=Stiffness_Buffer_Push_FL
  Sum : Sum  Inputs=|-+
  Push Force : Outport  InitialOutput=0  VectorParamsAs1DForOutWhenUnconnected=off
  wires:
  length/1 -> Sum/1
  Stiffness_Push/1 -> Push Force/1
  Sum/1 -> Stiffness_Push/1
  Constant/1 -> Sum/2

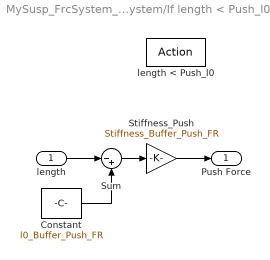
== system MySusp_FrcSystem_RTW/MySusp_FrcSystem/MySusp_BufferSystem/If length < Push_l0 FR ==
  length : Inport
  length < Push_l0 : ActionPort  ActionPortLabel=if(u1 < l0_Buffer_Push_FR)
  Constant : Constant  Value=l0_Buffer_Push_FR
  Stiffness_Push : Gain  Gain=Stiffness_Buffer_Push_FR
  Sum : Sum  Inputs=|-+
  Push Force : Outport  InitialOutput=0  VectorParamsAs1DForOutWhenUnconnected=off
  wires:
  length/1 -> Sum/1
  Stiffness_Push/1 -> Push Force/1
  Sum/1 -> Stiffness_Push/1
  Constant/1 -> Sum/2

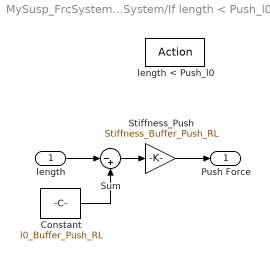
== system MySusp_FrcSystem_RTW/MySusp_FrcSystem/MySusp_BufferSystem/If length < Push_l0 RL ==
  length : Inport
  length < Push_l0 : ActionPort  ActionPortLabel=if(u1 < l0_Buffer_Push_RL)
  Constant : Constant  Value=l0_Buffer_Push_RL
  Stiffness_Push : Gain  Gain=Stiffness_Buffer_Push_RL
  Sum : Sum  Inputs=|-+
  Push Force : Outport  InitialOutput=0  VectorParamsAs1DForOutWhenUnconnected=off
  wires:
  length/1 -> Sum/1
  Stiffness_Push/1 -> Push Force/1
  Sum/1 -> Stiffness_Push/1
  Constant/1 -> Sum/2

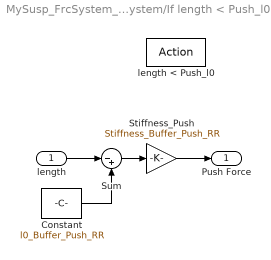
== system MySusp_FrcSystem_RTW/MySusp_FrcSystem/MySusp_BufferSystem/If length < Push_l0 RR ==
  length : Inport
  length < Push_l0 : ActionPort  ActionPortLabel=if(u1 < l0_Buffer_Push_RR)
  Constant : Constant  Value=l0_Buffer_Push_RR
  Stiffness_Push : Gain  Gain=Stiffness_Buffer_Push_RR
  Sum : Sum  Inputs=|-+
  Push Force : Outport  InitialOutput=0  VectorParamsAs1DForOutWhenUnconnected=off
  wires:
  length/1 -> Sum/1
  Stiffness_Push/1 -> Push Force/1
  Sum/1 -> Stiffness_Push/1
  Constant/1 -> Sum/2

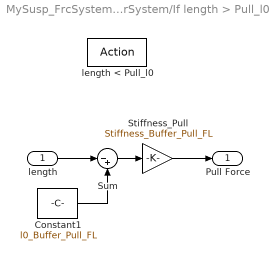
== system MySusp_FrcSystem_RTW/MySusp_FrcSystem/MySusp_BufferSystem/If length > Pull_l0 FL ==
  length : Inport
  length < Pull_l0 : ActionPort  ActionPortLabel=elseif(u1 > l0_Buffer_Pull_FL)
  Constant1 : Constant  Value=l0_Buffer_Pull_FL
  "Stiffness_Pull " : Gain  Gain=Stiffness_Buffer_Pull_FL
  Sum : Sum  Inputs=|-+
  Pull Force : Outport  InitialOutput=0  VectorParamsAs1DForOutWhenUnconnected=off
  wires:
  "Stiffness_Pull "/1 -> Pull Force/1
  Sum/1 -> "Stiffness_Pull "/1
  Constant1/1 -> Sum/2
  length/1 -> Sum/1

== system MySusp_FrcSystem_RTW/MySusp_FrcSystem/MySusp_BufferSystem/If length > Pull_l0 FR ==
  length : Inport
  length < Pull_l0 : ActionPort  ActionPortLabel=elseif(u1 > l0_Buffer_Pull_FR)
  Constant1 : Constant  Value=l0_Buffer_Pull_FR
  "Stiffness_Pull " : Gain  Gain=Stiffness_Buffer_Pull_FR
  Sum : Sum  Inputs=|-+
  Pull Force : Outport  InitialOutput=0  VectorParamsAs1DForOutWhenUnconnected=off
  wires:
  "Stiffness_Pull "/1 -> Pull Force/1
  Sum/1 -> "Stiffness_Pull "/1
  Constant1/1 -> Sum/2
  length/1 -> Sum/1

== system MySusp_FrcSystem_RTW/MySusp_FrcSystem/MySusp_BufferSystem/If length > Pull_l0 RL ==
  length : Inport
  length < Pull_l0 : ActionPort  ActionPortLabel=elseif(u1 > l0_Buffer_Pull_RL)
  Constant1 : Constant  Value=l0_Buffer_Pull_RL
  "Stiffness_Pull " : Gain  Gain=Stiffness_Buffer_Pull_RL
  Sum : Sum  Inputs=|-+
  Pull Force : Outport  InitialOutput=0  VectorParamsAs1DForOutWhenUnconnected=off
  wires:
  "Stiffness_Pull "/1 -> Pull Force/1
  Sum/1 -> "Stiffness_Pull "/1
  Constant1/1 -> Sum/2
  length/1 -> Sum/1

== system MySusp_FrcSystem_RTW/MySusp_FrcSystem/MySusp_BufferSystem/If length > Pull_l0 RR ==
  length : Inport
  length < Pull_l0 : ActionPort  ActionPortLabel=elseif(u1 > l0_Buffer_Pull_RR)
  Constant1 : Constant  Value=l0_Buffer_Pull_RR
  "Stiffness_Pull " : Gain  Gain=Stiffness_Buffer_Pull_RR
  Sum : Sum  Inputs=|-+
  Pull Force : Outport  InitialOutput=0  VectorParamsAs1DForOutWhenUnconnected=off
  wires:
  "Stiffness_Pull "/1 -> Pull Force/1
  Sum/1 -> "Stiffness_Pull "/1
  Constant1/1 -> Sum/2
  length/1 -> Sum/1
